simulink model "Lab3"  (R2023b)
settings: Solver=FixedStepAuto  StartTime=0.0  StopTime=10000.0  FixedStep=0.1  RelTol=1e-3
values from neighbouring files (symbols this model uses):
  a = 1    [Lab3_driver.m]
  a1 = 1    [Lab3_driver.m]
  b = 2    [Lab3_driver.m]
  K = 4    [Lab3_driver.m]
  mu = 0    [Lab3_driver.m]
  n = 10    [Lab3_driver.m]
  p = 0.1    [Lab3_driver.m]
  sigma = 1    [Lab3_driver.m]
libraries: dspmathops x1
settings Model: PauseTimes=1  Creator=alberto  LastModifiedBy=alberto

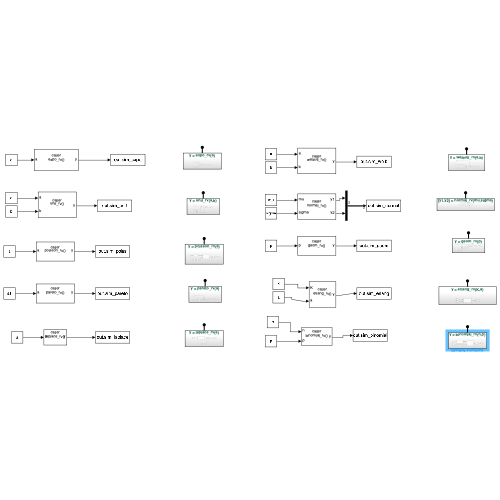
[thumbnail: Simulink's stored preview of the top-level diagram]
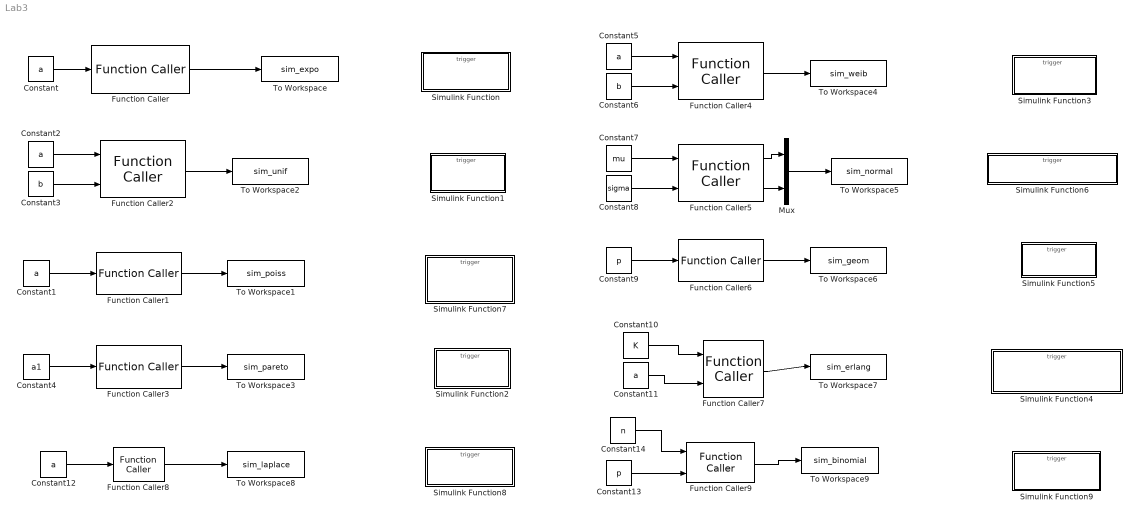
== system Lab3 ==
  Constant{,1..2,5,11..12} (6 alike) : Constant  Value=a  SampleTime=-1
  Constant10 : Constant  Value=K
  Constant13 : Constant  Value=p  SampleTime=-1
  Constant14 : Constant  Value=n
  Constant3 : Constant  Value=b  SampleTime=-1
  Constant4 : Constant  Value=a1  SampleTime=-1
  Constant6 : Constant  Value=b  SampleTime=-1
  Constant7 : Constant  Value=mu  SampleTime=-1
  Constant8 : Constant  Value=sigma  SampleTime=-1
  Constant9 : Constant  Value=p  SampleTime=-1
  Function Caller : FunctionCaller  FunctionPrototype=y = expo_rv(a)
  Function Caller1 : FunctionCaller  FunctionPrototype=y = poisson_rv(a)  InputArgumentSpecifications=<Enter example>  OutputArgumentSpecifications=<Enter example>
  Function Caller2 : FunctionCaller  FunctionPrototype=y = unif_rv(a,b)  InputArgumentSpecifications=<Enter example>  OutputArgumentSpecifications=<Enter example>
  Function Caller3 : FunctionCaller  FunctionPrototype=y = pareto_rv(a)  InputArgumentSpecifications=<Enter example>  OutputArgumentSpecifications=<Enter example>
  Function Caller4 : FunctionCaller  FunctionPrototype=y = weibull_rv(a,b)  InputArgumentSpecifications=<Enter example>  OutputArgumentSpecifications=<Enter example>
  Function Caller5 : FunctionCaller  FunctionPrototype=[y1,y2] = normal_rv(mu,sigma)  InputArgumentSpecifications=<Enter example>  OutputArgumentSpecifications=<Enter example>
  Function Caller6 : FunctionCaller  FunctionPrototype=y = geom_rv(p)  InputArgumentSpecifications=<Enter example>  OutputArgumentSpecifications=<Enter example>
  Function Caller7 : FunctionCaller  FunctionPrototype=y = erlang_rv(K,a)  InputArgumentSpecifications=<Enter example>  OutputArgumentSpecifications=<Enter example>
  Function Caller8 : FunctionCaller  FunctionPrototype=y = laplace_rv(a)  InputArgumentSpecifications=<Enter example>  OutputArgumentSpecifications=<Enter example>
  Function Caller9 : FunctionCaller  FunctionPrototype=y = binomial_rv(n,p)  InputArgumentSpecifications=<Enter example>  OutputArgumentSpecifications=<Enter example>
  Mux : Mux  Inputs=2
  Simulink Function : Subsystem  TreatAsAtomicUnit=on
  Simulink Function1 : Subsystem  TreatAsAtomicUnit=on
  Simulink Function2 : Subsystem  TreatAsAtomicUnit=on
  Simulink Function3 : Subsystem  TreatAsAtomicUnit=on
  Simulink Function4 : Subsystem  TreatAsAtomicUnit=on
  Simulink Function5 : Subsystem  TreatAsAtomicUnit=on
  Simulink Function6 : Subsystem  TreatAsAtomicUnit=on
  Simulink Function7 : Subsystem  TreatAsAtomicUnit=on
  Simulink Function8 : Subsystem  TreatAsAtomicUnit=on
  Simulink Function9 : Subsystem  TreatAsAtomicUnit=on
  To Workspace : ToWorkspace  VariableName=sim_expo  SaveFormat=Timeseries  SampleTime=-1
  To Workspace1 : ToWorkspace  VariableName=sim_poiss  SaveFormat=Timeseries  SampleTime=-1
  To Workspace2 : ToWorkspace  VariableName=sim_unif  SaveFormat=Timeseries  SampleTime=-1
  To Workspace3 : ToWorkspace  VariableName=sim_pareto  SaveFormat=Timeseries  SampleTime=-1
  To Workspace4 : ToWorkspace  VariableName=sim_weib  SaveFormat=Timeseries  SampleTime=-1
  To Workspace5 : ToWorkspace  VariableName=sim_normal  SaveFormat=Timeseries  SampleTime=-1
  To Workspace6 : ToWorkspace  VariableName=sim_geom  SaveFormat=Timeseries  SampleTime=-1
  To Workspace7 : ToWorkspace  VariableName=sim_erlang  SaveFormat=Timeseries  SampleTime=-1
  To Workspace8 : ToWorkspace  VariableName=sim_laplace  SaveFormat=Timeseries  SampleTime=-1
  To Workspace9 : ToWorkspace  VariableName=sim_binomial  SaveFormat=Timeseries  SampleTime=-1
  wires:
  Constant/1 -> Function Caller/1
  Function Caller/1 -> To Workspace/1
  Constant1/1 -> Function Caller1/1
  Function Caller1/1 -> To Workspace1/1
  Constant2/1 -> Function Caller2/1
  Constant3/1 -> Function Caller2/2
  Function Caller2/1 -> To Workspace2/1
  Function Caller3/1 -> To Workspace3/1
  Constant4/1 -> Function Caller3/1
  Constant6/1 -> Function Caller4/2
  Function Caller4/1 -> To Workspace4/1
  Constant5/1 -> Function Caller4/1
  Constant8/1 -> Function Caller5/2
  Function Caller5/1 -> Mux/1
  Constant7/1 -> Function Caller5/1
  Constant9/1 -> Function Caller6/1
  Function Caller6/1 -> To Workspace6/1
  Function Caller5/2 -> Mux/2
  Mux/1 -> To Workspace5/1
  Constant10/1 -> Function Caller7/1
  Constant11/1 -> Function Caller7/2
  Function Caller7/1 -> To Workspace7/1
  Constant12/1 -> Function Caller8/1
  Function Caller8/1 -> To Workspace8/1
  Constant13/1 -> Function Caller9/2
  Function Caller9/1 -> To Workspace9/1
  Constant14/1 -> Function Caller9/1

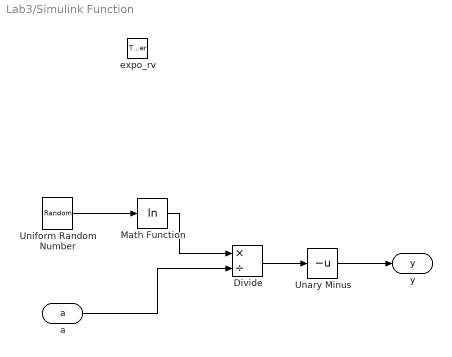
== system Lab3/Simulink Function ==
  expo_rv : TriggerPort  TriggerType=function-call  IsSimulinkFunction=on  FunctionName=expo_rv  FunctionVisibility=scoped  VariantControl=(inherit)
  Divide : Product  Inputs=*/
  Math Function : Math  Operator=log
  Unary Minus : UnaryMinus
  Uniform Random Number : UniformRandomNumber  Minimum=0  VectorParams1D=off
  a : ArgIn  DisableCoverage=on  ArgumentName=a
  y : ArgOut  DisableCoverage=on  ArgumentName=y
  wires:
  a/1 -> Divide/2
  Uniform Random Number/1 -> Math Function/1
  Math Function/1 -> Divide/1
  Divide/1 -> Unary Minus/1
  Unary Minus/1 -> y/1

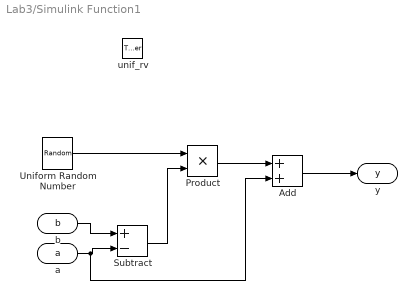
== system Lab3/Simulink Function1 ==
  unif_rv : TriggerPort  TriggerType=function-call  IsSimulinkFunction=on  FunctionName=unif_rv  FunctionVisibility=scoped  VariantControl=(inherit)
  Add : Sum
  Product : Product
  Subtract : Sum  Inputs=+-
  Uniform Random Number : UniformRandomNumber  Minimum=0
  a : ArgIn  DisableCoverage=on  ArgumentName=a
  b : ArgIn  Port=2  ArgumentName=b
  y : ArgOut  DisableCoverage=on  ArgumentName=y
  wires:
  a/1 -> Add/2, Subtract/2
  b/1 -> Subtract/1
  Subtract/1 -> Product/2
  Uniform Random Number/1 -> Product/1
  Product/1 -> Add/1
  Add/1 -> y/1

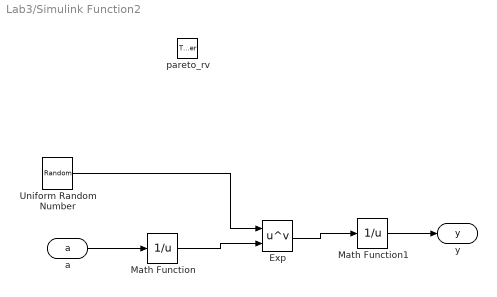
== system Lab3/Simulink Function2 ==
  pareto_rv : TriggerPort  TriggerType=function-call  IsSimulinkFunction=on  FunctionName=pareto_rv  FunctionVisibility=scoped  VariantControl=(inherit)
  Exp : Math  Operator=pow
  Math Function : Math  Operator=reciprocal
  Math Function1 : Math  Operator=reciprocal
  Uniform Random Number : UniformRandomNumber  Minimum=0
  a : ArgIn  DisableCoverage=on  ArgumentName=a
  y : ArgOut  DisableCoverage=on  ArgumentName=y
  wires:
  Uniform Random Number/1 -> Exp/1
  Exp/1 -> Math Function1/1
  Math Function1/1 -> y/1
  a/1 -> Math Function/1
  Math Function/1 -> Exp/2

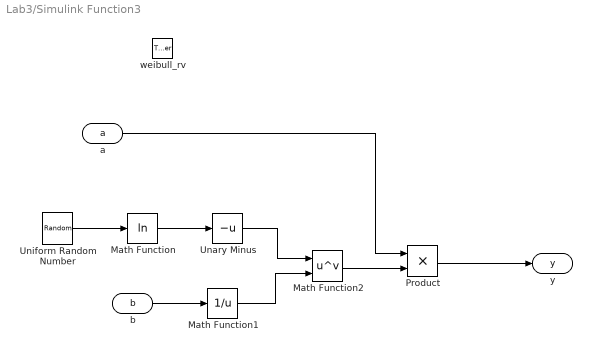
== system Lab3/Simulink Function3 ==
  weibull_rv : TriggerPort  TriggerType=function-call  IsSimulinkFunction=on  FunctionName=weibull_rv  FunctionVisibility=scoped  VariantControl=(inherit)
  Math Function : Math  Operator=log
  Math Function1 : Math  Operator=reciprocal
  Math Function2 : Math  Operator=pow
  Product : Product
  Unary Minus : UnaryMinus
  Uniform Random Number : UniformRandomNumber  Minimum=0
  a : ArgIn  DisableCoverage=on  ArgumentName=a
  b : ArgIn  Port=2  ArgumentName=b
  y : ArgOut  DisableCoverage=on  ArgumentName=y
  wires:
  a/1 -> Product/1
  Uniform Random Number/1 -> Math Function/1
  b/1 -> Math Function1/1
  Math Function/1 -> Unary Minus/1
  Unary Minus/1 -> Math Function2/1
  Math Function1/1 -> Math Function2/2
  Math Function2/1 -> Product/2
  Product/1 -> y/1

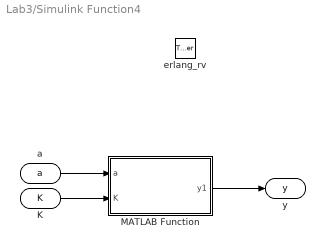
== system Lab3/Simulink Function4 ==
  erlang_rv : TriggerPort  TriggerType=function-call  IsSimulinkFunction=on  FunctionName=erlang_rv  FunctionVisibility=scoped  VariantControl=(inherit)
  MATLAB Function : MATLAB Function  TreatAsAtomicUnit=on
  K : ArgIn  DisableCoverage=on  ArgumentName=K
  a : ArgIn  Port=2  ArgumentName=a
  y : ArgOut  DisableCoverage=on  ArgumentName=y
  wires:
  MATLAB Function/1(y1) -> y/1
  a/1 -> MATLAB Function/1(a)
  K/1 -> MATLAB Function/2(K)

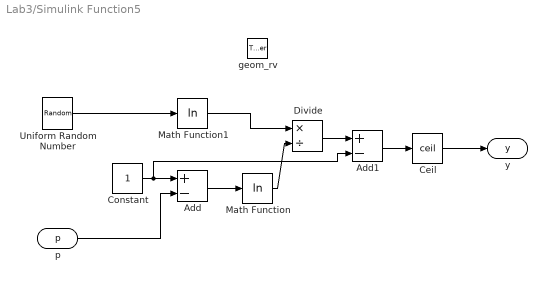
== system Lab3/Simulink Function5 ==
  geom_rv : TriggerPort  TriggerType=function-call  IsSimulinkFunction=on  FunctionName=geom_rv  FunctionVisibility=scoped  VariantControl=(inherit)
  Add : Sum  Inputs=+-
  Add1 : Sum  Inputs=+-
  Ceil : Rounding  Operator=ceil
  Constant : Constant
  Divide : Product  Inputs=*/
  Math Function : Math  Operator=log
  Math Function1 : Math  Operator=log
  Uniform Random Number : UniformRandomNumber  Minimum=0  Seed=randi(456782)
  p : ArgIn  DisableCoverage=on  ArgumentName=p
  y : ArgOut  DisableCoverage=on  ArgumentName=y
  wires:
  p/1 -> Add/2
  Constant/1 -> Add1/2, Add/1
  Add/1 -> Math Function/1
  Uniform Random Number/1 -> Math Function1/1
  Math Function1/1 -> Divide/1
  Math Function/1 -> Divide/2
  Divide/1 -> Add1/1
  Add1/1 -> Ceil/1
  Ceil/1 -> y/1

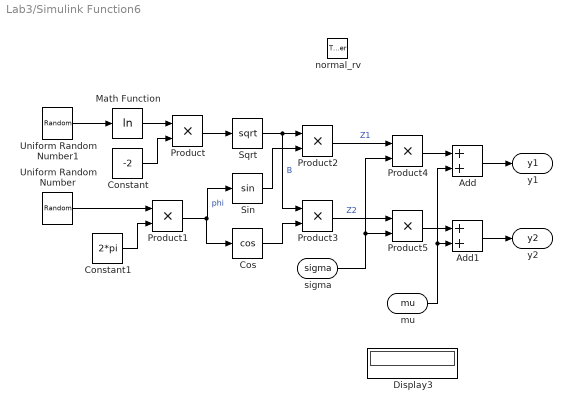
== system Lab3/Simulink Function6 ==
  normal_rv : TriggerPort  TriggerType=function-call  IsSimulinkFunction=on  FunctionName=normal_rv  FunctionVisibility=scoped  VariantControl=(inherit)
  Add : Sum
  Add1 : Sum
  Constant : Constant  Value=-2
  Constant1 : Constant  Value=2*pi
  Cos : Trigonometry  Operator=cos
  Display3 : Display
  Math Function : Math  Operator=log
  Product{,1..5} (6 alike) : Product
  Sin : Trigonometry
  Sqrt : Sqrt
  Uniform Random Number : UniformRandomNumber  Minimum=0  Seed=randi(1000)
  Uniform Random Number1 : UniformRandomNumber  Minimum=0  Seed=randi(1000)
  mu : ArgIn  DisableCoverage=on  ArgumentName=mu
  sigma : ArgIn  Port=2  ArgumentName=sigma
  y1 : ArgOut  DisableCoverage=on  ArgumentName=y1
  y2 : ArgOut  Port=2  ArgumentName=y2
  wires:
  mu/1 -> Add/2, Add1/2
  Uniform Random Number1/1 -> Math Function/1
  Math Function/1 -> Product/1
  Constant/1 -> Product/2
  Product/1 -> Sqrt/1
  Uniform Random Number/1 -> Product1/1
  Constant1/1 -> Product1/2
  Product1/1 -> Cos/1, Sin/1  "phi"
  Sqrt/1 -> Product3/1, Product2/1  "B"
  Sin/1 -> Product2/2
  Cos/1 -> Product3/2
  Product2/1 -> Product4/1  "Z1"
  Product3/1 -> Product5/1  "Z2"
  sigma/1 -> Product5/2, Product4/2
  Product4/1 -> Add/1
  Product5/1 -> Add1/1
  Add/1 -> y1/1
  Add1/1 -> y2/1

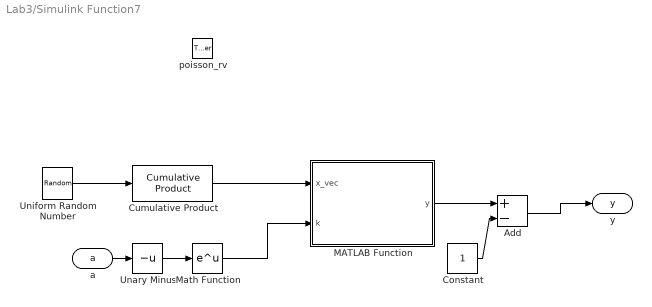
== system Lab3/Simulink Function7 ==
  poisson_rv : TriggerPort  TriggerType=function-call  IsSimulinkFunction=on  FunctionName=poisson_rv  FunctionVisibility=scoped  VariantControl=(inherit)
  Add : Sum  Inputs=+-
  Constant : Constant
  Cumulative Product : dspmathops/Cumulative Product  dim=Columns  InputProcessing=Columns as channels (frame based)  reset_popup=None  roundingMode=Floor  overflowMode=off  outputMin=[]  outputMax=[]
  MATLAB Function : MATLAB Function  TreatAsAtomicUnit=on
  Math Function : Math
  Unary Minus : UnaryMinus
  Uniform Random Number : UniformRandomNumber  Minimum=zeros(100,1)  Maximum=ones(100,1)  Seed=randi(10000,100,1)  VectorParams1D=off
  a : ArgIn  DisableCoverage=on  ArgumentName=a
  y : ArgOut  DisableCoverage=on  ArgumentName=y
  wires:
  a/1 -> Unary Minus/1
  Uniform Random Number/1 -> Cumulative Product/1
  Unary Minus/1 -> Math Function/1
  Math Function/1 -> MATLAB Function/2(k)
  Cumulative Product/1 -> MATLAB Function/1(x_vec)
  MATLAB Function/1(y) -> Add/1
  Constant/1 -> Add/2
  Add/1 -> y/1

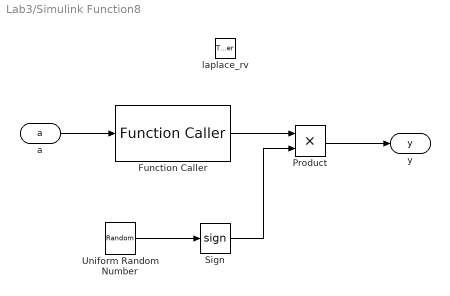
== system Lab3/Simulink Function8 ==
  laplace_rv : TriggerPort  TriggerType=function-call  IsSimulinkFunction=on  FunctionName=laplace_rv  FunctionVisibility=scoped  VariantControl=(inherit)
  Function Caller : FunctionCaller  FunctionPrototype=y = expo_rv(a)
  Product : Product
  Sign : Signum
  Uniform Random Number : UniformRandomNumber
  a : ArgIn  DisableCoverage=on  ArgumentName=a
  y : ArgOut  DisableCoverage=on  ArgumentName=y
  wires:
  a/1 -> Function Caller/1
  Function Caller/1 -> Product/1
  Uniform Random Number/1 -> Sign/1
  Sign/1 -> Product/2
  Product/1 -> y/1

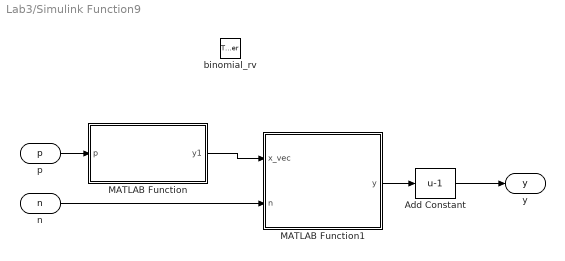
== system Lab3/Simulink Function9 ==
  binomial_rv : TriggerPort  TriggerType=function-call  IsSimulinkFunction=on  FunctionName=binomial_rv  FunctionVisibility=scoped  VariantControl=(inherit)
  Add Constant : Bias  Bias=-1  SaturateOnIntegerOverflow=off
  MATLAB Function : MATLAB Function  TreatAsAtomicUnit=on
  MATLAB Function1 : MATLAB Function  TreatAsAtomicUnit=on
  n : ArgIn  DisableCoverage=on  ArgumentName=n
  p : ArgIn  Port=2  ArgumentName=p
  y : ArgOut  DisableCoverage=on  ArgumentName=y
  wires:
  p/1 -> MATLAB Function/1(p)
  MATLAB Function/1(y1) -> MATLAB Function1/1(x_vec)
  n/1 -> MATLAB Function1/2(n)
  MATLAB Function1/1(y) -> Add Constant/1
  Add Constant/1 -> y/1

== matlab function Lab3/Simulink Function7/MATLAB Function ==
  data: x_vec input; y output; k input
function y = first_index_lower(x_vec, k)


y = zeros(1);
y(1) = find(x_vec < k, 1, 'first');

== matlab function Lab3/Simulink Function9/MATLAB Function ==
  data: p input; y1 output
function y1 = geometric_cumsum(p)

y1 = zeros(100,1);
app_var = zeros(100,1);
for ind = 1:100
    app_var(ind) = geom_rv(p);
end
y1 = cumsum(app_var);

== matlab function Lab3/Simulink Function9/MATLAB Function1 ==
  data: x_vec input; y output; n input
function y = first_index_larger(x_vec, n)


y = zeros(1);
y(1) = find(x_vec > n, 1, 'first');

== matlab function Lab3/Simulink Function4/MATLAB Function ==
  data: y1 output; a input; K input
function y1 = expo_rv_caller(a, K)

y1 = 0;
for ind = 1:K
    y1 = y1 + expo_rv(a);
end
